simulink model "FirstOrderSystemImpulseResponse"  (R2017b)
settings: Solver=VariableStepAuto  StartTime=0.0  StopTime=1  RelTol=1e-3
undefined symbols (not defined in the file): sigma
libraries: dspsrcs4 x1
settings Model: Creator=Riz  LastModifiedBy=Riz

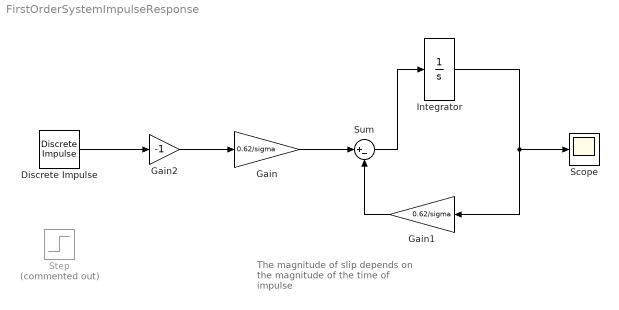
== system FirstOrderSystemImpulseResponse ==
  note: The magnitude of slip depends
      | on the magnitude of the time of
      | impulse
  Discrete Impulse : dspsrcs4/Discrete  Impulse  Delay=0  SampleTime=1e-5  FrameSample=1  OutputFrames=off  dataType=double  isSigned=on  wordLen=16  udDataType=sfix(16)  fracBitsMode=Best precision  numFracBits=15  OutDataTypeStr=double  LastOutDataTypeStr=double
  Gain : Gain  Gain=0.62/sigma
  Gain1 : Gain  Gain=0.62/sigma
  Gain2 : Gain  Gain=-1
  Integrator : Integrator
  Scope : Scope
  Step : Step  Commented=on  Time=0  SampleTime=0
  Sum : Sum  Inputs=|+-
  wires:
  Gain/1 -> Sum/1
  Sum/1 -> Integrator/1
  Integrator/1 -> Scope/1, Gain1/1
  Gain1/1 -> Sum/2
  Gain2/1 -> Gain/1
  Discrete Impulse/1 -> Gain2/1
